simulink model "ctrl_custom"  (R2016b)
settings: Solver=ode3  StartTime=0.0  StopTime=inf  FixedStep=0.01  RelTol=1e-3  EnableMultiTasking=on
undefined symbols (not defined in the file): C, D, DiscIntNeverNeededParam, eps_c, epsilon, hd, hd2, I_s, k_cc, K_omega, K_q1f, K_q1r, K_q2f, K_q2r, K_q3f, K_q3r, K_q4f, K_q4r, K_q5f, K_q5r, K_q6f, K_q6r, K_T1f, K_T1r, K_T2f, K_T2r, K_T3f, K_T3r, K_T4f, K_T4r, K_T5f, K_T5r, K_T6f, K_T6r, Kp, Max_Acceleration, Max_rotation, Max_thrust, Min_thrust, n_c, n_max, p_cc, pwm_thr1_backward, pwm_thr1_forward, pwm_thr2_backward, pwm_thr2_forward, pwm_thr3_backward, pwm_thr3_forward, pwm_thr4_backward, pwm_thr4_forward, pwm_thr5_backward, pwm_thr5_forward, pwm_thr6_backward, pwm_thr6_forward, Q_f0, Q_max, r_cc, Rho, Thruster
libraries: dspmtrx3 x10, marine_gnc x9, simulink x7, simulink_extras x3
(part 5 of 5)

== system ctrl_custom/Thruster control /Thruster 6/Thruster control/Core controller ==
  note: Core controller: Shaft speed
  n_r : Inport
  "Tr " : Inport  Port=2
  "n " : Inport  Port=3
  Core controller: Torque,Power and Combined Torque/Power : MATLAB Function  TreatAsAtomicUnit=on
  Integrator : Integrator  ExternalReset=either  UpperSaturationLimit=Q_max  LowerSaturationLimit=-Q_max
  Ki : Gain  Gain=Kp/0.05
  Kp : Gain  Gain=Kp
  Sum : Sum  Inputs=+|-
  Sum1 : Sum  Inputs=|++
  reset : S-Function  Priority=1  FunctionName=NIVeriStandIO  Parameters=width dtype portnum stime stype btype  SFunctionDeploymentMode=off  EnableBusSupport=off  mask(NI VeriStand Inport){portnum=1, width=-1, stime=-1, dtype=auto, stype=auto, btype=1}
      mask prompts: portnum "Port number:"; width "Port dimensions (-1 for dynamically sized):"; stime "Sample time (-1 for inherited):"; dtype "Data type:"; stype "Signal type:"; btype "Block type:"
      mask help: Use this inport on any level of nested subsystems to allow NI VeriStand software to map signals to it.
      mask init:
      | NIVeriStandIO_init;
      settings: CopyFcn=NIVeriStand_MDL_functions('', 'IO_copy');  DeleteFcn=NIVeriStand_MDL_functions('', 'IO_delete');  MoveFcn=set_param(gcb, 'Mask', 'on');
      mask Callback portnum: NIVeriStand_MDL_functions('', 'IO_setportnum');
      mask TypeOptions dtype: auto | double | single | int8 | uint8 | int16 | uint16 | int32 | uint32 | boolean
      mask Callback dtype: NIVeriStand_MDL_functions('', 'IO_booleansignal');
      mask TypeOptions stype: auto | real | complex
      mask Display:
      | patch([-x x], [-y y], [.90980 .81960 .32156]);
      | plot([xrad -x x xrad], [yrad -y y yrad]);
      | fprintf('NI In%d', portnum);
  Q_cn : Outport
  Qcq : Outport  Port=2
  Qcp : Outport  Port=3
  Qcc : Outport  Port=4
  wires:
  n_r/1 -> Sum/1
  Ki/1 -> Integrator/1
  Kp/1 -> Sum1/1
  Integrator/1 -> Sum1/2
  Sum/1 -> Ki/1, Kp/1
  Sum1/1 -> Q_cn/1
  reset/1 -> Integrator/2
  [k_cc] -> Core controller: Torque,Power and Combined Torque/Power/1(k_cc)
  [p_cc] -> Core controller: Torque,Power and Combined Torque/Power/2(p_cc)
  [r_cc] -> Core controller: Torque,Power and Combined Torque/Power/3(r_cc)
  Core controller: Torque,Power and Combined Torque/Power/3(Qcc) -> Qcc/1
  [Kt6f] -> Core controller: Torque,Power and Combined Torque/Power/5(K_t0)
  [D] -> Core controller: Torque,Power and Combined Torque/Power/7(D)
  [Kq6f] -> Core controller: Torque,Power and Combined Torque/Power/6(K_q0)
  [Rho] -> Core controller: Torque,Power and Combined Torque/Power/9(rho)
  "n "/1 -> Core controller: Torque,Power and Combined Torque/Power/4(n), Sum/2
  "Tr "/1 -> Core controller: Torque,Power and Combined Torque/Power/8(Tr)
  Core controller: Torque,Power and Combined Torque/Power/2(Qcp) -> Qcp/1
  Core controller: Torque,Power and Combined Torque/Power/1(Qcq) -> Qcq/1
  [eps_c] -> Core controller: Torque,Power and Combined Torque/Power/10(eps_c)
  [Kt6r] -> Core controller: Torque,Power and Combined Torque/Power/11(K_t0r)
  [Kq6r] -> Core controller: Torque,Power and Combined Torque/Power/12(K_q0r)

== matlab function ctrl_custom/Referance/MATLAB Function ==
  data: omega input; y output; zeta input
function y = fcn(omega,zeta)

y = 2*zeta*omega;

== matlab function ctrl_custom/Referance/MATLAB Function1 ==
  data: omega input; y output; zeta input
function y = fcn(omega,zeta)

y = 2*zeta*omega;

== matlab function ctrl_custom/Referance/MATLAB Function2 ==
  data: omega input; y output
function y = fcn(omega)

y = omega*omega;

== matlab function ctrl_custom/Thrust allocation/Optimal angle path and constraints on rotation speed/Ensuring angle is [-pi pi] ==
  data: angle input; y output
function y = rad2pipi(angle)
% RAD2PIPI Converts an angle in rad to the interval (-pi pi]
%          Should be applied to all heading errors in a feedback control system
%          in order to avoid discontinuities.
%
% Author:     Roger Skjetne
% Date:       2003-09-05
% Revisions:  2004-09-02 Thor I. Fossen - replaced input argument x with angle
%             2005-01-05 Thor I. Fossen - ouput argument is set to y and not angle
%             2005-04-13 Roger Skjetne  - changed the function s in order
%                                         to account for correct mapping to
%                                         (-pi pi].
%
% ________________________________________________________________
%
% MSS GNC is a Matlab toolbox for guidance, navigation and control.
% The toolbox is part of the Marine Systems Simulator (MSS).
%
% Copyright (C) 2008 Thor I. Fossen and Tristan Perez
% 
% This program is free software: you can redistribute it and/or modify
% it under the terms of the GNU General Public License as published by
% the Free Software Foundation, either version 3 of the License, or
% (at your option) any later version.
% 
% This program is distributed in the hope that it will be useful, but
% WITHOUT ANY WARRANTY; without even the implied warranty of
% MERCHANTABILITY or FITNESS FOR A PARTICULAR PURPOSE.  See the 
% GNU General Public License for more details.
% 
% You should have received a copy of the GNU General Public License
% along with this program.  If not, see <http://www.gnu.org/licenses/>.
% 
% E-mail: contact@marinecontrol.org
% URL:    <http://www.marinecontrol.org>


% convert angle in rad to the interval <-pi pi> 
r = rem(angle+sign(angle)*pi,2*pi);
s = sign(sign(angle) + 2*(sign(abs(rem(angle+pi,2*pi)/(2*pi)))-1));
% s = sign(angle);

y = r - s*pi;

== matlab function ctrl_custom/Thruster control /Thrust and Shaft speed mapped to PWM/MATLAB Function1 ==
  data: Tc_in1 input; signal input; Tc_out output; Tc_in2 input
function Tc_out = fcn(Tc_in1,signal,Tc_in2)
%#codegen

if signal >= 0
    Tc_out = Tc_in1;
else %signal < 0
    Tc_out = Tc_in2;
end

== matlab function ctrl_custom/Thrust allocation/Optimal angle path and constraints on rotation speed/MATLAB Function1 ==
  data: desired input; psi_D output; actual input
function psi_D   = fcn(desired,actual)
%#codegen
psi_D = desired-actual;
if abs(psi_D) >= 360
    psi_D = rem(psi_D,360);
end

if abs(psi_D) >= 180
    psi_D = psi_D - sign(psi_D)*360;
end

% if desired < 0 %&& abs(desired+actual) > 180
%     y = actual+360;
% else
%     y = abs(actual);
% end

%if desired-actual > 180
%    u = desired - 360;
%elseif desired-actual <= -180
%    u=actual + 360 ;
%else
%    u=desired;        
%end

end

%rotation = change-actual;% - actual; % If positive with clock, Negative against clock
%if rotation >= 180 || rotation <= -180
% u = desired;
%else 
%     u = actual;
%end

%change = abs(actual);

% if actual-desired > 180 && desired > 0 && rotation > 0
%     u = -180;
% elseif  actual-desired > 180 && desired > 0 && rotation < 0
%     u = 180;
% else 
%     u = actual;
% end

% if change > abs(desired-actual)
%     u = -actual;
% else
%     u = actual;
% end
% if desired >= 0.98*actual || desired <= -0.98*actual 
%     u = desired;
% else 
%     u = actual; 
% end
% paths = [abs(actual-desired),abs(-1*actual-desired)];
% fastest = min(paths);
% if paths(1) > paths(2)
%     fastest = paths(2);
% elseif paths(1) < paths(2)
%     fastest = paths(1);
% end
% % if desired > 0 && actual < 0 || desired < 0 && actual < 0
% % u = fastest;
% % elseif desired > 0 && actual > 0 || desired < 0 && actual < 0
% %     u = fastest;
% if desired-actual > 180 || desired-actual < -180
%     u = -actual;
% else 
%     u = actual;
% end

== matlab function ctrl_custom/Thrust allocation/MATLAB Function ==
  data: u input; sys output; ThrusterPosX input; ThrusterPosY input; C input
function sys = fcn(u,ThrusterPosX,ThrusterPosY,C)
% Complete system goes here!
Alpha1 = zeros(1,6);    % Allocating dimensions for faster computing
% Parameters thrusters
tc =  [u(1),u(2),u(3)]'; 
alpha = [u(4),u(5),u(6),u(7),u(8),u(9)]';

% Constraints for Thruster-Thruster interaction. Can be seen in "Initfile"
% how they are found
C1 = C(1,:);
C2 = C(2,:);
C3 = C(3,:);
C4 = C(4,:);
C5 = C(5,:);
C6 = C(6,:);

K = ones(1,6);

K = ones(1,6);

if alpha(1) < C1(1)-0.1  && alpha(1) > C1(2)+0.1 || alpha(1) > C1(3)+0.1 && alpha(1) < C1(4)-0.1
    K(1) = 0;
else 
    K(1) = K(1);
end

if alpha(2) > C2(1)-0.1  && alpha(2) < C2(2)+0.1 || alpha(2) > C2(3)-0.1 && alpha(2) < C2(4)+0.1
    K(2) = 0;
else 
    K(2) = K(2);
end

if alpha(3) < C3(1)+0.1  && alpha(3) > C3(2)-0.1 || alpha(3) < C3(3)+0.1 && alpha(3) > C3(4)-0.1
    K(3) = 0;
else 
    K(3) = K(3);
end

if alpha(4) > C4(1)+0.1  && alpha(4) < C4(2)-0.1 || alpha(4) < C4(3)-0.1 && alpha(4) > C4(4)+0.1
    K(4) = 0;
else 
    K(4) = K(4);
end

if alpha(5) < C5(1)-0.1  && alpha(5) > C5(2)+0.1 || alpha(5) < C5(3)-0.1 && alpha(5) > C5(4)+0.1
    K(5) = 0;
else 
    K(5) = K(5);
end

if alpha(6) > C6(1)+0.1  && alpha(6) < C6(2)-0.1 || alpha(6) > C6(3)+0.1 && alpha(6) < C6(4)-0.1
    K(6) = 0;
else 
    K(6) = K(6);
end

epsilon = u(10);

n_t = length(ThrusterPosX); % number of thrusters
B_surge = zeros(n_t,1); % Shells for faster computing
B_sway = zeros(n_t,1);  % Shells for faster computing
B_yaw = zeros(n_t,1);   % Shells for faster computing

for i = 1:1:n_t
  B_surge(i) = cosd(alpha(i));     %Thrust in x-direction for cartesian
  B_sway(i) = sind(alpha(i));      %Thrust in y-direction for cartesian
  B_yaw(i) = (sind(alpha(i))*ThrusterPosX(i) - cosd(alpha(i))*ThrusterPosY(i));
end


B = [B_surge,B_sway,B_yaw]';
B = B*diag(K); 
[U_singular,S_singular,V_singular] = svd(B,'econ');
S_singular_cross = 1./S_singular;
S_singular_cross(~isfinite(S_singular_cross))=0;
 if (S_singular_cross(3,3)>10*S_singular_cross(2,2)) 
     S_singular_cross(3,3)=0;
 end
 
u_optimized = V_singular*S_singular_cross*U_singular';

u_d = u_optimized*tc;          % Optimized Thrust



Te = [1 0 1 0 1 0 1 0 1 0 1 0;
      0 1 0 1 0 1 0 1 0 1 0 1;
      ThrusterPosY(1) ThrusterPosX(1) ThrusterPosY(2) ThrusterPosX(2) ThrusterPosY(3) ThrusterPosX(3) ...
      ThrusterPosY(4) ThrusterPosX(4) ThrusterPosY(5) ThrusterPosX(5) ThrusterPosY(6) ThrusterPosX(6)];

[U_singular,S_singular,V_singular] = svd(Te,'econ');
S_singular_cross = 1./S_singular;
S_singular_cross(~isfinite(S_singular_cross))=0;
 if (S_singular_cross(3,3)>2*S_singular_cross(2,2)) 
     S_singular_cross(3,3)=0;
 end
T0 = V_singular*S_singular_cross*U_singular'*tc;

alpha1 = [atan2d(T0(2),T0(1)) atan2d(T0(4),T0(3)) atan2d(T0(6),T0(5)) atan2d(T0(8),T0(7)) atan2d(T0(10),T0(9)) atan2d(T0(12),T0(11))];


%% Constraints
% Thruster 1 OK
%C1 = [151 130 -151 -130 ];
if alpha1(1) < C1(1)  && alpha1(1) > C1(2) && u_d(1) > 0 || alpha1(1) < C1(1)  && alpha1(1) > C1(2) && u_d(1) < 0
    c1 = [C1(1) C1(2)];
    [C_1,alpha_new1] = min(abs(c1-alpha1(1)));
    Alpha1(1) = c1(alpha_new1);
elseif alpha1(1) > C1(3) && alpha1(1) < C1(4) && u_d(1) > 0 || alpha1(1) > C1(3) && alpha1(1) < C1(4) && u_d(1) < 0
    c1 = [C1(3) C1(4)];
    [C_1,alpha_new1] = min(abs(c1-alpha1(1)));
    Alpha1(1) = c1(alpha_new1);
else 
    Alpha1(1) = alpha1(1);
end
if alpha(1) < C1(1)-0.1  && alpha(1) > C1(2)+0.1 || alpha(1) > C1(3)+0.1 && alpha(1) < C1(4)-0.1
    u_d(1) = 0;
else 
    u_d(1) = u_d(1);
end

% Thruster 2 
%C2 = [-99.85 -80.15 -50 -29];
if alpha1(2) < C2(1)  && alpha1(2) > C2(2) && u_d(2) > 0 || alpha1(2) < C2(1)  && alpha1(2) > C2(2) && u_d(2) < 0 
    c2 = [C2(1) C2(2)];
    [C_2,alpha_new2] = min(abs(c2-alpha1(2)));
    Alpha1(2) = c2(alpha_new2);
elseif alpha1(2) < C2(3) && alpha1(2) > C2(4) && u_d(2) > 0 || alpha1(2) < C2(3) && alpha1(2) > C2(4) && u_d(2) < 0
    c2 = [C2(3) C2(4)];
    [C_2,alpha_new2] = min(abs(c2-alpha1(2)));
    Alpha1(2) = c2(alpha_new2);
else 
    Alpha1(2) = alpha1(2);
end
if alpha(2) < C2(1)-0.1  && alpha(2) > C2(2)+0.1 || alpha(2) < C2(3)-0.1 && alpha(2) > C2(4)+0.1
    u_d(2) = 0;
else 
    u_d(2) = u_d(2);
end

% Thruster 3 
% C3 = [99.85 80.15 50 29]; 

if alpha1(3) > C3(1)  && alpha1(3) < C3(2) && u_d(3) > 0 || alpha1(3) > C3(1)  && alpha1(3) < C3(2) && u_d(3) < 0
    c3 = [C3(1) C3(2)];
    [C_3,alpha_new3] = min(abs(c3-alpha1(3)));
    Alpha1(3) = c3(alpha_new3);
elseif alpha1(3) > C3(3) && alpha1(3) < C3(4) && u_d(3) > 0 || alpha1(3) > C3(3) && alpha1(3) < C3(4) && u_d(3) < 0 
    c3 = [C3(3) C3(4)];
    [C_3,alpha_new3] = min(abs(c3-alpha1(3)));
    Alpha1(3) = c3(alpha_new3);
else 
    Alpha1(3) = alpha1(3);
end
if alpha(3) > C3(1)+0.1  && alpha(3) < C3(2)-0.1 || alpha(3) > C3(3)+0.1 && alpha(3) < C3(4)-0.1
    u_d(3) = 0;
else 
    u_d(3) = u_d(3);
end

% Thruster 4 OK
%C4 = [-52.8 -34.2 52.8 34.2]; 
if alpha1(4) > C4(1)  && alpha1(4) < C4(2) && u_d(4) > 0 || alpha1(4) > C4(1)  && alpha1(4) < C4(2) && u_d(4) < 0
    c4 = [C4(1) C4(2)];
    [C_4,alpha_new4] = min(abs(c4-alpha1(4)));
    Alpha1(4) = c4(alpha_new4);
elseif alpha1(4) < C4(3) && alpha1(4) > C4(4) && u_d(4) > 0 || alpha1(4) < C4(3) && alpha1(4) > C4(4) && u_d(4) < 0 
    c4 = [C4(3) C4(4)];
    [C_4,alpha_new4] = min(abs(c4-alpha1(4)));
    Alpha1(4) = c4(alpha_new4);
else 
    Alpha1(4) = alpha1(4);
end
if alpha(4) > C4(1)+0.1  && alpha(4) < C4(2)-0.1 || alpha(4) < C4(3)-0.1 && alpha(4) > C4(4)+0.1
    u_d(4) = 0;
else 
    u_d(4) = u_d(4);
end

% Thruster 5
%C5 = [-98.25 -81.75 -145.8 -127.2];
if alpha1(5) < C5(1)  && alpha1(5) > C5(2) && u_d(5) > 0 || alpha1(5) < C5(1)  && alpha1(5) > C5(2) && u_d(5) < 0
    c5 = [C5(1) C5(2)];
    [C_5,alpha_new5] = min(abs(c5-alpha1(5)));
    Alpha1(5) = c5(alpha_new5);
elseif alpha1(5) < C5(3) && alpha1(5) > C5(4) && u_d(5) > 0  || alpha1(5) < C5(3) && alpha1(5) > C5(4) && u_d(5) < 0
    c5 = [C5(3) C5(4)];
    [C_5,alpha_new5] = min(abs(c5-alpha1(5)));
    Alpha1(5) = c5(alpha_new5);
else 
    Alpha1(5) = alpha1(5);
end
if alpha(5) < C5(1)-0.1  && alpha(5) > C5(2)+0.1 || alpha(5) < C5(3)-0.1 && alpha(5) > C5(4)+0.1
    u_d(5) = 0;
else 
    u_d(5) = u_d(5);
end

% Thruster 6
%C6 = [98.75 81.75 145.8 127.2];
if alpha1(6) > C6(1)  && alpha1(6) < C6(2) && u_d(6) > 0 || alpha1(6) > C6(1)  && alpha1(6) < C6(2) && u_d(6) < 0
    c6 = [C6(1) C6(2)];
    [C_6,alpha_new6] = min(abs(c6-alpha1(6)));
    Alpha1(6) = c6(alpha_new6);
elseif alpha1(6) > C6(3) && alpha1(6) < C6(4) && u_d(6) > 0 || alpha1(6) > C6(3) && alpha1(6) < C6(4) && u_d(6) < 0
    c6 = [C6(3) C6(4)];
    [C_6,alpha_new6] = min(abs(c6-alpha1(6)));
    Alpha1(6) = c6(alpha_new6);
else 
    Alpha1(6) = alpha1(6);
end
if alpha(6) > C6(1)+0.1  && alpha(6) < C6(2)-0.1 || alpha(6) > C6(3)+0.1 && alpha(6) < C6(4)-0.1
    u_d(6) = 0;
else 
    u_d(6) = u_d(6);
end

% Thruster 2&3 
if Alpha1(2) == C2(2)
    Alpha1(3) = alpha1(2) - (C2(2) - alpha1(2));
elseif Alpha1(2) == C2(1)
    Alpha1(3) = alpha1(2) - (C2(1) - alpha1(2));
elseif Alpha1(2) == C2(3)
    Alpha1(3) = alpha1(2) - (C2(3) - alpha1(2));
elseif Alpha1(2) == C2(4)
    Alpha1(3) = alpha1(2) - (C2(4) - alpha1(2));
    
elseif Alpha1(3) == C3(2)
    Alpha1(2) = alpha1(3) - (C3(2) - alpha1(3));
elseif Alpha1(3) == C3(1)
    Alpha1(2) = alpha1(3) - (C3(1) - alpha1(3));
elseif Alpha1(3) == C3(3)
    Alpha1(2) = alpha1(3) - (C3(3) - alpha1(3));
elseif Alpha1(3) == C3(4)
    Alpha1(2) = alpha1(3) - (C3(4) - alpha1(3));
end

% Thruster 5&6
if Alpha1(5) == C5(2)
    Alpha1(6) = alpha1(5) - (C5(2) - alpha1(5));
elseif Alpha1(5) == C5(1)
    Alpha1(6) = alpha1(5) - (C5(1) - alpha1(5));
elseif Alpha1(5) == C5(3)
    Alpha1(6) = alpha1(5) - (C5(3) - alpha1(5));
elseif Alpha1(5) == C5(4)
    Alpha1(6) = alpha1(5) - (C5(4) - alpha1(5));
    
elseif Alpha1(6) == C6(2)
    Alpha1(5) = alpha1(6) - (C6(2) - alpha1(6));
elseif Alpha1(6) == C6(1)
    Alpha1(5) = alpha1(6) - (C6(1) - alpha1(6));
elseif Alpha1(6) == C6(3)
    Alpha1(5) = alpha1(6) - (C6(3) - alpha1(6));
elseif Alpha1(6) == C6(4)
    Alpha1(5) = alpha1(6) - (C6(4) - alpha1(6));
end
% Thruster 4 & 1
if     Alpha1(4) == C4(2)
    Alpha1(1) = alpha1(4) - (C4(2) - alpha1(4));
elseif Alpha1(4) == C4(1)
    Alpha1(1) = alpha1(4) - (C4(1) - alpha1(4));
elseif Alpha1(4) == C4(3)
    Alpha1(1) = alpha1(4) - (C4(3) - alpha1(4));
elseif Alpha1(4) == C4(4)
    Alpha1(1) = alpha1(4) - (C4(4) - alpha1(4));
end

if     Alpha1(1) == C1(2)
    Alpha1(4) = alpha1(1) - (C1(2) - alpha1(1));
elseif Alpha1(1) == C1(1)
    Alpha1(4) = alpha1(1) - (C1(1) - alpha1(1));
elseif Alpha1(1) == C1(3)
    Alpha1(4) = alpha1(1) - (C1(3) - alpha1(1));
elseif Alpha1(1) == C1(4)
    Alpha1(4) = alpha1(1) - (C1(4) - alpha1(1));
end

Alpha1 = [Alpha1(1) Alpha1(2) Alpha1(3) Alpha1(4) Alpha1(5) Alpha1(6)]';    
Desired_thrust = [u_d(1) u_d(2) u_d(3) u_d(4) u_d(5) u_d(6)]';
alpha_desired = Alpha1;


% u_d = -Desired_thrust;
%% Update outputs
sys = [alpha_desired',u_d']';

== matlab function ctrl_custom/Thruster control /Thruster 1/Propeller Hydrodynamics/Actual Force and Torque ==
  data: Ta output; n input; Qa output; Kq input; Kt input; Ktr input; Kqr input; Rho input; D input; eps_c input; env input; Pa output
function [Ta,Qa,Pa]= ActualForces(n,Kq,Kt,Ktr,Kqr,Rho,D,eps_c,env)
%#codegen
lambda_c = 0.5+0.5*tanh(eps_c*n/5); % Smooth switching between positive and negative thrust. 5 makes switch happen between -5 and 5
K_TC = Kt*lambda_c+(1-lambda_c)*Ktr;
K_QC = Kq*lambda_c+(1-lambda_c)*Kqr;

Ta = sign(n)*K_TC*Rho*(D^4)*n^2-env;
Qa = sign(n)*K_QC*Rho*(D^5)*n^2-env;
Pa = 2*pi*n*Qa;

== matlab function ctrl_custom/Thruster control /Thruster 1/Thruster control/MATLAB Function ==
  data: Td input; n_d output; K_t0 input; K_t0r input; rho input; D input; eps_c input; n_c input; n_r input; T_r output
function [n_d,T_r]  = ReferenceGenerator(Td,K_t0,K_t0r,rho,D,eps_c,n_c,n_r)
%#codegen


n_d = sign(Td)*sqrt((abs(Td))/(rho*D^4*K_t0));

lambda_c = 0.5+0.5*tanh(eps_c*n_d/5); % Smooth switching between positive and negative thrust. 5 makes switch happen between -5 and 5
K_TC = K_t0*lambda_c+(1-lambda_c)*K_t0r;

T_r = sign(n_r)*K_TC*rho*D^4*n_r^2;

== matlab function ctrl_custom/Thruster control /Thruster 1/Thruster control/Supervisor ==
  data: control input; input input; n input; u output
function u = fcn(control,input,n)
u = 1;
if control == 1
if input == 1
    u = 1;
elseif input == 2
    u = 2;
elseif input == 3 && n > 0 || input == 3 && n < 0
    u = 3;
elseif input == 4 || input == 3 && n == 0
    u = 4;
else 
    u = 5;
end
end

if control == 2
if input == 1
    u = 1;
elseif input == 2
    u = 2;
elseif input == 3 && n > 0 || input == 3 && n < 0
    u = 3;
elseif input == 4 || input == 3 && n == 0
    u = 4;
else 
    u = 5;
end
end

if control == 3
if input == 1
    u = 1;
elseif input == 2
    u = 2;
elseif input == 3 && n > 0 || input == 3 && n < 0
    u = 3;
elseif input == 4 || input == 3 && n == 0
    u = 4;
else 
    u = 5;
end
end

if control == 4
if input == 1
    u = 1;
elseif input == 2
    u = 2;
elseif input == 3 && n > 0 || input == 3 && n < 0
    u = 3;
elseif input == 4 || input == 3 && n == 0
    u = 4;
else 
    u = 5;
end
end

if control == 5
if input == 1
    u = 1;
elseif input == 2
    u = 2;
elseif input == 3 && n > 0 || input == 3 && n < 0
    u = 3;
elseif input == 4 || input == 3 && n == 0
    u = 4;
else 
    u = 5;
end
end

== matlab function ctrl_custom/Thruster control /Thruster 1/Thruster control/Core controller/Core controller: Torque,Power and Combined Torque//Power ==
  data: Qcq output; Qcp output; k_cc input; p_cc input; r_cc input; n input; Qcc output; K_t0 input; K_q0 input; D input; Tr input; rho input; eps_c input; K_t0r input; K_q0r input
function [Qcq,Qcp,Qcc]= CoreControl(k_cc,p_cc,r_cc,n,K_t0,K_q0,D,Tr,rho,eps_c,K_t0r,K_q0r)
%#codegen

lambda_c = 0.5+0.5*tanh(eps_c*n/5);
K_TC = K_t0*lambda_c+(1-lambda_c)*K_t0r;
K_QC = K_q0*lambda_c+(1-lambda_c)*K_q0r;
Qcq = (K_QC/K_TC)*D*Tr;
if n == 0
    Qcp = 0;
else
Qcp = sign(Tr)*K_QC*(abs(Tr)^(3/2))/(sqrt(rho)*D*K_TC^(3/2)*abs(n));
end
alpha_c = exp(-k_cc*abs(p_cc*n)^r_cc);

Qcc = alpha_c*Qcq + (1-alpha_c)*Qcp;

== matlab function ctrl_custom/Thruster control /Thrust and Shaft speed mapped to PWM/MATLAB Function2 ==
  data: Tc_in1 input; signal input; Tc_out output; Tc_in2 input
function Tc_out = fcn(Tc_in1,signal,Tc_in2)
%#codegen

if signal >= 0
    Tc_out = Tc_in1;
else %signal < 0
    Tc_out = Tc_in2;
end

== matlab function ctrl_custom/Thruster control /Thruster 2/Propeller Hydrodynamics/Actual Force and Torque ==
  data: Ta output; n input; Qa output; Kq input; Kt input; Ktr input; Kqr input; Rho input; D input; eps_c input; env input
function [Ta,Qa]= ActualForces(n,Kq,Kt,Ktr,Kqr,Rho,D,eps_c,env)
%#codegen
lambda_c = 0.5+0.5*tanh(eps_c*n/5); % Smooth switching between positive and negative thrust. 5 makes switch happen between -5 and 5
K_TC = Kt*lambda_c+(1-lambda_c)*Ktr;
K_QC = Kq*lambda_c+(1-lambda_c)*Kqr;

Ta = sign(n)*K_TC*Rho*(D^4)*n^2-env;
Qa = sign(n)*K_QC*Rho*(D^5)*n^2-env;

== matlab function ctrl_custom/Initialization of parameters/Guidance Gains/MATLAB Function ==
  data: T_x input; y output
function y = fcn(T_x)

y = 1/T_x;

== matlab function ctrl_custom/Thrust allocation/angle between [-180 180] ==
  data: angle input; y output
function y = rad2pipi(angle)
% RAD2PIPI Converts an angle in rad to the interval (-pi pi]
%          Should be applied to all heading errors in a feedback control system
%          in order to avoid discontinuities.
%
% Author:     Roger Skjetne
% Date:       2003-09-05
% Revisions:  2004-09-02 Thor I. Fossen - replaced input argument x with angle
%             2005-01-05 Thor I. Fossen - ouput argument is set to y and not angle
%             2005-04-13 Roger Skjetne  - changed the function s in order
%                                         to account for correct mapping to
%                                         (-pi pi].
%
% ________________________________________________________________
%
% MSS GNC is a Matlab toolbox for guidance, navigation and control.
% The toolbox is part of the Marine Systems Simulator (MSS).
%
% Copyright (C) 2008 Thor I. Fossen and Tristan Perez
% 
% This program is free software: you can redistribute it and/or modify
% it under the terms of the GNU General Public License as published by
% the Free Software Foundation, either version 3 of the License, or
% (at your option) any later version.
% 
% This program is distributed in the hope that it will be useful, but
% WITHOUT ANY WARRANTY; without even the implied warranty of
% MERCHANTABILITY or FITNESS FOR A PARTICULAR PURPOSE.  See the 
% GNU General Public License for more details.
% 
% You should have received a copy of the GNU General Public License
% along with this program.  If not, see <http://www.gnu.org/licenses/>.
% 
% E-mail: contact@marinecontrol.org
% URL:    <http://www.marinecontrol.org>


% convert angle in rad to the interval <-pi pi> 
r = rem(angle+sign(angle)*pi,2*pi);
s = sign(sign(angle) + 2*(sign(abs(rem(angle+pi,2*pi)/(2*pi)))-1));
% s = sign(angle);

y = r - s*pi;

== matlab function ctrl_custom/Initialization of parameters/Guidance Gains/MATLAB Function1 ==
  data: T_y input; y output
function y = fcn(T_y)

y = 1/T_y;

== matlab function ctrl_custom/Initialization of parameters/Guidance Gains/MATLAB Function2 ==
  data: T_psi input; y output
function y = fcn(T_psi)

y = 1/T_psi;

== matlab function ctrl_custom/Thruster control /Thrust and Shaft speed mapped to PWM/MATLAB Function3 ==
  data: Tc_in1 input; signal input; Tc_out output; Tc_in2 input
function Tc_out = fcn(Tc_in1,signal,Tc_in2)
%#codegen

if signal >= 0
    Tc_out = Tc_in1;
else %signal < 0
    Tc_out = Tc_in2;
end

== matlab function ctrl_custom/Thruster control /Thruster 2/Thruster control/Core controller/Core controller: Torque,Power and Combined Torque//Power ==
  data: Qcq output; Qcp output; k_cc input; p_cc input; r_cc input; n input; Qcc output; K_t0 input; K_q0 input; D input; Tr input; rho input; eps_c input; K_t0r input; K_q0r input
function [Qcq,Qcp,Qcc]= CoreControl(k_cc,p_cc,r_cc,n,K_t0,K_q0,D,Tr,rho,eps_c,K_t0r,K_q0r)
%#codegen

lambda_c = 0.5+0.5*tanh(eps_c*n/5);
K_TC = K_t0*lambda_c+(1-lambda_c)*K_t0r;
K_QC = K_q0*lambda_c+(1-lambda_c)*K_q0r;
Qcq = (K_QC/K_TC)*D*Tr;
if n == 0
    Qcp = 0;
else
Qcp = sign(Tr)*K_QC*(abs(Tr)^(3/2))/(sqrt(rho)*D*K_TC^(3/2)*abs(n));
end
alpha_c = exp(-k_cc*abs(p_cc*n)^r_cc);

Qcc = alpha_c*Qcq + (1-alpha_c)*Qcp;

== matlab function ctrl_custom/Thruster control /Thruster 2/Thruster control/MATLAB Function ==
  data: Td input; n_d output; K_t0 input; K_t0r input; rho input; D input; eps_c input; n_c input; n_r input; T_r output
function [n_d,T_r]  = ReferenceGenerator(Td,K_t0,K_t0r,rho,D,eps_c,n_c,n_r)
%#codegen


n_d = sign(Td)*sqrt((abs(Td))/(rho*D^4*K_t0));

lambda_c = 0.5+0.5*tanh(eps_c*n_d/5); % Smooth switching between positive and negative thrust
K_TC = K_t0*lambda_c+(1-lambda_c)*K_t0r;

T_r = sign(n_r)*K_TC*rho*D^4*n_r^2;

== matlab function ctrl_custom/Thruster control /Thruster 2/Thruster control/Supervisor ==
  data: control input; input input; n input; u output
function u = fcn(control,input,n)
u = 1;
if control == 1
if input == 1
    u = 1;
elseif input == 2
    u = 2;
elseif input == 3 && n > 0 || input == 3 && n < 0
    u = 3;
elseif input == 4 || input == 3 && n == 0
    u = 4;
else 
    u = 5;
end
end

if control == 2
if input == 1
    u = 1;
elseif input == 2
    u = 2;
elseif input == 3 && n > 0 || input == 3 && n < 0
    u = 3;
elseif input == 4 || input == 3 && n == 0
    u = 4;
else 
    u = 5;
end
end

if control == 3
if input == 1
    u = 1;
elseif input == 2
    u = 2;
elseif input == 3 && n > 0 || input == 3 && n < 0
    u = 3;
elseif input == 4 || input == 3 && n == 0
    u = 4;
else 
    u = 5;
end
end

if control == 4
if input == 1
    u = 1;
elseif input == 2
    u = 2;
elseif input == 3 && n > 0 || input == 3 && n < 0
    u = 3;
elseif input == 4 || input == 3 && n == 0
    u = 4;
else 
    u = 5;
end
end

if control == 5
if input == 1
    u = 1;
elseif input == 2
    u = 2;
elseif input == 3 && n > 0 || input == 3 && n < 0
    u = 3;
elseif input == 4 || input == 3 && n == 0
    u = 4;
else 
    u = 5;
end
end

== matlab function ctrl_custom/Thruster control /Thrust and Shaft speed mapped to PWM/MATLAB Function4 ==
  data: Tc_in1 input; signal input; Tc_out output; Tc_in2 input
function Tc_out = fcn(Tc_in1,signal,Tc_in2)
%#codegen

if signal >= 0
    Tc_out = Tc_in1;
else %signal < 0
    Tc_out = Tc_in2;
end

== matlab function ctrl_custom/Thruster control /Thruster 3/Propeller Hydrodynamics/Actual Force and Torque ==
  data: Ta output; n input; Qa output; Kq input; Kt input; Ktr input; Kqr input; Rho input; D input; eps_c input; env input
function [Ta,Qa]= ActualForces(n,Kq,Kt,Ktr,Kqr,Rho,D,eps_c,env)
%#codegen
lambda_c = 0.5+0.5*tanh(eps_c*n/5); % Smooth switching between positive and negative thrust. 5 makes switch happen between -5 and 5
K_TC = Kt*lambda_c+(1-lambda_c)*Ktr;
K_QC = Kq*lambda_c+(1-lambda_c)*Kqr;

Ta = sign(n)*K_TC*Rho*(D^4)*n^2-env;
Qa = sign(n)*K_QC*Rho*(D^5)*n^2-env;

== matlab function ctrl_custom/MATLAB Function ==
  data: thrust_actual input; commanded_tau output; alpha_actual input; PosX input; PosY input
function commanded_tau   = fcn(thrust_actual,alpha_actual,PosX,PosY)
%#codegen

Alpha_surge =[cosd(alpha_actual(1)) cosd(alpha_actual(2)) cosd(alpha_actual(3)) cosd(alpha_actual(4)) cosd(alpha_actual(5)) cosd(alpha_actual(6))];  
Alpha_sway = [sind(alpha_actual(1)) sind(alpha_actual(2)) sind(alpha_actual(3)) sind(alpha_actual(4)) sind(alpha_actual(5)) sind(alpha_actual(6))];
Alpha_yaw = [sind(alpha_actual(1))*PosX(1)-cosd(alpha_actual(1))*PosY(1) sind(alpha_actual(2))*PosX(2)-cosd(alpha_actual(2))*PosY(2) ...
             sind(alpha_actual(3))*PosX(3)-cosd(alpha_actual(3))*PosY(3) sind(alpha_actual(4))*PosX(4)-cosd(alpha_actual(4))*PosY(4) ...
             sind(alpha_actual(5))*PosX(5)-cosd(alpha_actual(5))*PosY(5) sind(alpha_actual(6))*PosX(6)-cosd(alpha_actual(6))*PosY(6)];

commanded_tau = [Alpha_surge;Alpha_sway;Alpha_yaw]*thrust_actual;

== matlab function ctrl_custom/Thruster control /Thrust and Shaft speed mapped to PWM/MATLAB Function5 ==
  data: Tc_in1 input; signal input; Tc_out output; Tc_in2 input
function Tc_out = fcn(Tc_in1,signal,Tc_in2)
%#codegen

if signal >= 0
    Tc_out = Tc_in1;
else %signal < 0
    Tc_out = Tc_in2;
end

== matlab function ctrl_custom/Thruster control /Thruster 3/Thruster control/Core controller/Core controller: Torque,Power and Combined Torque//Power ==
  data: Qcq output; Qcp output; k_cc input; p_cc input; r_cc input; n input; Qcc output; K_t0 input; K_q0 input; D input; Tr input; rho input; eps_c input; K_t0r input; K_q0r input
function [Qcq,Qcp,Qcc]= CoreControl(k_cc,p_cc,r_cc,n,K_t0,K_q0,D,Tr,rho,eps_c,K_t0r,K_q0r)
%#codegen

lambda_c = 0.5+0.5*tanh(eps_c*n/5);
K_TC = K_t0*lambda_c+(1-lambda_c)*K_t0r;
K_QC = K_q0*lambda_c+(1-lambda_c)*K_q0r;
Qcq = (K_QC/K_TC)*D*Tr;
if n == 0
    Qcp = 0;
else
Qcp = sign(Tr)*K_QC*(abs(Tr)^(3/2))/(sqrt(rho)*D*K_TC^(3/2)*abs(n));
end
alpha_c = exp(-k_cc*abs(p_cc*n)^r_cc);

Qcc = alpha_c*Qcq + (1-alpha_c)*Qcp;

== matlab function ctrl_custom/Thruster control /Thruster 3/Thruster control/MATLAB Function ==
  data: Td input; n_d output; K_t0 input; K_t0r input; rho input; D input; eps_c input; n_c input; n_r input; T_r output
function [n_d,T_r]  = ReferenceGenerator(Td,K_t0,K_t0r,rho,D,eps_c,n_c,n_r)
%#codegen


n_d = sign(Td)*sqrt((abs(Td))/(rho*D^4*K_t0));

lambda_c = 0.5+0.5*tanh(eps_c*n_d/5); % Smooth switching between positive and negative thrust
K_TC = K_t0*lambda_c+(1-lambda_c)*K_t0r;

T_r = sign(n_r)*K_TC*rho*D^4*n_r^2;

== matlab function ctrl_custom/Thruster control /Thrust and Shaft speed mapped to PWM/MATLAB Function ==
  data: input input; output output; control input; speedcontrol input
function output = fcn(input,control,speedcontrol)
%#codegen
if control == 1
output = [input(1) speedcontrol(1) input(3) speedcontrol(2) input(5) speedcontrol(3) input(7) speedcontrol(4) input(9) speedcontrol(5) input(11) speedcontrol(6)]';
%     output = [input(1) input(2) input(3) input(4) input(5) input(6) input(7) input(8) input(9) input(10) input(11) input(12)]';

else
    output = [input(1) input(2) input(3) input(4) input(5) input(6) input(7) input(8) input(9) input(10) input(11) input(12)]';

end

== matlab function ctrl_custom/Thruster control /Thrust and Shaft speed mapped to PWM/MATLAB Function6 ==
  data: Tc_in1 input; signal input; Tc_out output; Tc_in2 input
function Tc_out = fcn(Tc_in1,signal,Tc_in2)
%#codegen

if signal >= 0
    Tc_out = Tc_in1;
else %signal < 0
    Tc_out = Tc_in2;
end

== matlab function ctrl_custom/Initialization of parameters/Setpoint Chasing/MATLAB Function ==
  data: Ts_x input; y output
function y = fcn(Ts_x)

Ts_x_model = Ts_x/sqrt(90);

y = 1/Ts_x_model;

== matlab function ctrl_custom/Initialization of parameters/Setpoint Chasing/MATLAB Function1 ==
  data: Ts_y input; y output
function y = fcn(Ts_y)

Ts_y_model = Ts_y/sqrt(90);

y = 1/Ts_y_model;

== matlab function ctrl_custom/Thruster control /Thruster 3/Thruster control/Supervisor ==
  data: control input; input input; n input; u output
function u = fcn(control,input,n)
u = 1;
if control == 1
if input == 1
    u = 1;
elseif input == 2
    u = 2;
elseif input == 3 && n > 0 || input == 3 && n < 0
    u = 3;
elseif input == 4 || input == 3 && n == 0
    u = 4;
else 
    u = 5;
end
end

if control == 2
if input == 1
    u = 1;
elseif input == 2
    u = 2;
elseif input == 3 && n > 0 || input == 3 && n < 0
    u = 3;
elseif input == 4 || input == 3 && n == 0
    u = 4;
else 
    u = 5;
end
end

if control == 3
if input == 1
    u = 1;
elseif input == 2
    u = 2;
elseif input == 3 && n > 0 || input == 3 && n < 0
    u = 3;
elseif input == 4 || input == 3 && n == 0
    u = 4;
else 
    u = 5;
end
end

if control == 4
if input == 1
    u = 1;
elseif input == 2
    u = 2;
elseif input == 3 && n > 0 || input == 3 && n < 0
    u = 3;
elseif input == 4 || input == 3 && n == 0
    u = 4;
else 
    u = 5;
end
end

if control == 5
if input == 1
    u = 1;
elseif input == 2
    u = 2;
elseif input == 3 && n > 0 || input == 3 && n < 0
    u = 3;
elseif input == 4 || input == 3 && n == 0
    u = 4;
else 
    u = 5;
end
end

== matlab function ctrl_custom/Thruster control /Thruster 4/Propeller Hydrodynamics/Actual Force and Torque ==
  data: Ta output; n input; Qa output; Kq input; Kt input; Ktr input; Kqr input; Rho input; D input; eps_c input; env input
function [Ta,Qa]= ActualForces(n,Kq,Kt,Ktr,Kqr,Rho,D,eps_c,env)
%#codegen
lambda_c = 0.5+0.5*tanh(eps_c*n/5); % Smooth switching between positive and negative thrust. 5 makes switch happen between -5 and 5
K_TC = Kt*lambda_c+(1-lambda_c)*Ktr;
K_QC = Kq*lambda_c+(1-lambda_c)*Kqr;

Ta = sign(n)*K_TC*Rho*(D^4)*n^2-env;
Qa = sign(n)*K_QC*Rho*(D^5)*n^2-env;

== matlab function ctrl_custom/Thruster control /Thruster 4/Thruster control/Core controller/Core controller: Torque,Power and Combined Torque//Power ==
  data: Qcq output; Qcp output; k_cc input; p_cc input; r_cc input; n input; Qcc output; K_t0 input; K_q0 input; D input; Tr input; rho input; eps_c input; K_t0r input; K_q0r input
function [Qcq,Qcp,Qcc]= CoreControl(k_cc,p_cc,r_cc,n,K_t0,K_q0,D,Tr,rho,eps_c,K_t0r,K_q0r)
%#codegen

lambda_c = 0.5+0.5*tanh(eps_c*n/5);
K_TC = K_t0*lambda_c+(1-lambda_c)*K_t0r;
K_QC = K_q0*lambda_c+(1-lambda_c)*K_q0r;
Qcq = (K_QC/K_TC)*D*Tr;
if n == 0
    Qcp = 0;
else
Qcp = sign(Tr)*K_QC*(abs(Tr)^(3/2))/(sqrt(rho)*D*K_TC^(3/2)*abs(n));
end
alpha_c = exp(-k_cc*abs(p_cc*n)^r_cc);

Qcc = alpha_c*Qcq + (1-alpha_c)*Qcp;

== matlab function ctrl_custom/Thruster control /Thruster 4/Thruster control/MATLAB Function ==
  data: Td input; n_d output; K_t0 input; K_t0r input; rho input; D input; eps_c input; n_c input; n_r input; T_r output
function [n_d,T_r]  = ReferenceGenerator(Td,K_t0,K_t0r,rho,D,eps_c,n_c,n_r)
%#codegen


n_d = sign(Td)*sqrt((abs(Td))/(rho*D^4*K_t0));

lambda_c = 0.5+0.5*tanh(eps_c*n_d/5); % Smooth switching between positive and negative thrust
K_TC = K_t0*lambda_c+(1-lambda_c)*K_t0r;

T_r = sign(n_r)*K_TC*rho*D^4*n_r^2;

== matlab function ctrl_custom/Thruster control /Thruster 4/Thruster control/Supervisor ==
  data: control input; input input; n input; u output
function u = fcn(control,input,n)
u = 1;
if control == 1
if input == 1
    u = 1;
elseif input == 2
    u = 2;
elseif input == 3 && n > 0 || input == 3 && n < 0
    u = 3;
elseif input == 4 || input == 3 && n == 0
    u = 4;
else 
    u = 5;
end
end

if control == 2
if input == 1
    u = 1;
elseif input == 2
    u = 2;
elseif input == 3 && n > 0 || input == 3 && n < 0
    u = 3;
elseif input == 4 || input == 3 && n == 0
    u = 4;
else 
    u = 5;
end
end

if control == 3
if input == 1
    u = 1;
elseif input == 2
    u = 2;
elseif input == 3 && n > 0 || input == 3 && n < 0
    u = 3;
elseif input == 4 || input == 3 && n == 0
    u = 4;
else 
    u = 5;
end
end

if control == 4
if input == 1
    u = 1;
elseif input == 2
    u = 2;
elseif input == 3 && n > 0 || input == 3 && n < 0
    u = 3;
elseif input == 4 || input == 3 && n == 0
    u = 4;
else 
    u = 5;
end
end

if control == 5
if input == 1
    u = 1;
elseif input == 2
    u = 2;
elseif input == 3 && n > 0 || input == 3 && n < 0
    u = 3;
elseif input == 4 || input == 3 && n == 0
    u = 4;
else 
    u = 5;
end
end

== matlab function ctrl_custom/Thruster control /Thruster 5/Propeller Hydrodynamics/Actual Force and Torque ==
  data: Ta output; n input; Qa output; Kq input; Kt input; Ktr input; Kqr input; Rho input; D input; eps_c input; env input
function [Ta,Qa]= ActualForces(n,Kq,Kt,Ktr,Kqr,Rho,D,eps_c,env)
%#codegen
lambda_c = 0.5+0.5*tanh(eps_c*n/5); % Smooth switching between positive and negative thrust. 5 makes switch happen between -5 and 5
K_TC = Kt*lambda_c+(1-lambda_c)*Ktr;
K_QC = Kq*lambda_c+(1-lambda_c)*Kqr;

Ta = sign(n)*K_TC*Rho*(D^4)*n^2-env;
Qa = sign(n)*K_QC*Rho*(D^5)*n^2-env;

== matlab function ctrl_custom/Thruster control /Thruster 5/Thruster control/Core controller/Core controller: Torque,Power and Combined Torque//Power ==
  data: Qcq output; Qcp output; k_cc input; p_cc input; r_cc input; n input; Qcc output; K_t0 input; K_q0 input; D input; Tr input; rho input; eps_c input; K_t0r input; K_q0r input
function [Qcq,Qcp,Qcc]= CoreControl(k_cc,p_cc,r_cc,n,K_t0,K_q0,D,Tr,rho,eps_c,K_t0r,K_q0r)
%#codegen

lambda_c = 0.5+0.5*tanh(eps_c*n/5);
K_TC = K_t0*lambda_c+(1-lambda_c)*K_t0r;
K_QC = K_q0*lambda_c+(1-lambda_c)*K_q0r;
Qcq = (K_QC/K_TC)*D*Tr;
if n == 0
    Qcp = 0;
else
Qcp = sign(Tr)*K_QC*(abs(Tr)^(3/2))/(sqrt(rho)*D*K_TC^(3/2)*abs(n));
end
alpha_c = exp(-k_cc*abs(p_cc*n)^r_cc);

Qcc = alpha_c*Qcq + (1-alpha_c)*Qcp;

== matlab function ctrl_custom/Thruster control /Thruster 5/Thruster control/MATLAB Function ==
  data: Td input; n_d output; K_t0 input; K_t0r input; rho input; D input; eps_c input; n_c input; n_r input; T_r output
function [n_d,T_r]  = ReferenceGenerator(Td,K_t0,K_t0r,rho,D,eps_c,n_c,n_r)
%#codegen


n_d = sign(Td)*sqrt((abs(Td))/(rho*D^4*K_t0));

lambda_c = 0.5+0.5*tanh(eps_c*n_d/5); % Smooth switching between positive and negative thrust
K_TC = K_t0*lambda_c+(1-lambda_c)*K_t0r;

T_r = sign(n_r)*K_TC*rho*D^4*n_r^2;

== matlab function ctrl_custom/Thruster control /Thruster 5/Thruster control/Supervisor ==
  data: control input; input input; n input; u output
function u = fcn(control,input,n)
u = 1;
if control == 1
if input == 1
    u = 1;
elseif input == 2
    u = 2;
elseif input == 3 && n > 0 || input == 3 && n < 0
    u = 3;
elseif input == 4 || input == 3 && n == 0
    u = 4;
else 
    u = 5;
end
end

if control == 2
if input == 1
    u = 1;
elseif input == 2
    u = 2;
elseif input == 3 && n > 0 || input == 3 && n < 0
    u = 3;
elseif input == 4 || input == 3 && n == 0
    u = 4;
else 
    u = 5;
end
end

if control == 3
if input == 1
    u = 1;
elseif input == 2
    u = 2;
elseif input == 3 && n > 0 || input == 3 && n < 0
    u = 3;
elseif input == 4 || input == 3 && n == 0
    u = 4;
else 
    u = 5;
end
end

if control == 4
if input == 1
    u = 1;
elseif input == 2
    u = 2;
elseif input == 3 && n > 0 || input == 3 && n < 0
    u = 3;
elseif input == 4 || input == 3 && n == 0
    u = 4;
else 
    u = 5;
end
end

if control == 5
if input == 1
    u = 1;
elseif input == 2
    u = 2;
elseif input == 3 && n > 0 || input == 3 && n < 0
    u = 3;
elseif input == 4 || input == 3 && n == 0
    u = 4;
else 
    u = 5;
end
end

== matlab function ctrl_custom/Thruster control /Thruster 6/Propeller Hydrodynamics/Actual Force and Torque ==
  data: Ta output; n input; Qa output; Kq input; Kt input; Ktr input; Kqr input; Rho input; D input; eps_c input; env input
function [Ta,Qa]= ActualForces(n,Kq,Kt,Ktr,Kqr,Rho,D,eps_c,env)
%#codegen
lambda_c = 0.5+0.5*tanh(eps_c*n/5); % Smooth switching between positive and negative thrust. 5 makes switch happen between -5 and 5
K_TC = Kt*lambda_c+(1-lambda_c)*Ktr;
K_QC = Kq*lambda_c+(1-lambda_c)*Kqr;

Ta = sign(n)*K_TC*Rho*(D^4)*n^2-env;
Qa = sign(n)*K_QC*Rho*(D^5)*n^2-env;

== matlab function ctrl_custom/Thruster control /Thruster 6/Thruster control/Core controller/Core controller: Torque,Power and Combined Torque//Power ==
  data: Qcq output; Qcp output; k_cc input; p_cc input; r_cc input; n input; Qcc output; K_t0 input; K_q0 input; D input; Tr input; rho input; eps_c input; K_t0r input; K_q0r input
function [Qcq,Qcp,Qcc]= CoreControl(k_cc,p_cc,r_cc,n,K_t0,K_q0,D,Tr,rho,eps_c,K_t0r,K_q0r)
%#codegen

lambda_c = 0.5+0.5*tanh(eps_c*n/5);
K_TC = K_t0*lambda_c+(1-lambda_c)*K_t0r;
K_QC = K_q0*lambda_c+(1-lambda_c)*K_q0r;
Qcq = (K_QC/K_TC)*D*Tr;
if n == 0
    Qcp = 0;
else
Qcp = sign(Tr)*K_QC*(abs(Tr)^(3/2))/(sqrt(rho)*D*K_TC^(3/2)*abs(n));
end
alpha_c = exp(-k_cc*abs(p_cc*n)^r_cc);

Qcc = alpha_c*Qcq + (1-alpha_c)*Qcp;

== matlab function ctrl_custom/Thruster control /Thruster 6/Thruster control/MATLAB Function ==
  data: Td input; n_d output; K_t0 input; K_t0r input; rho input; D input; eps_c input; n_c input; n_r input; T_r output
function [n_d,T_r]  = ReferenceGenerator(Td,K_t0,K_t0r,rho,D,eps_c,n_c,n_r)
%#codegen


n_d = sign(Td)*sqrt((abs(Td))/(rho*D^4*K_t0));

lambda_c = 0.5+0.5*tanh(eps_c*n_d/27); % Smooth switching between positive and negative thrust
K_TC = K_t0*lambda_c+(1-lambda_c)*K_t0r;

T_r = sign(n_r)*K_TC*rho*D^4*n_r^2;

== matlab function ctrl_custom/Thruster control /Thruster 6/Thruster control/Supervisor ==
  data: control input; input input; n input; u output
function u = fcn(control,input,n)
u = 1;
if control == 1
if input == 1
    u = 1;
elseif input == 2
    u = 2;
elseif input == 3 && n > 0 || input == 3 && n < 0
    u = 3;
elseif input == 4 || input == 3 && n == 0
    u = 4;
else 
    u = 5;
end
end

if control == 2
if input == 1
    u = 1;
elseif input == 2
    u = 2;
elseif input == 3 && n > 0 || input == 3 && n < 0
    u = 3;
elseif input == 4 || input == 3 && n == 0
    u = 4;
else 
    u = 5;
end
end

if control == 3
if input == 1
    u = 1;
elseif input == 2
    u = 2;
elseif input == 3 && n > 0 || input == 3 && n < 0
    u = 3;
elseif input == 4 || input == 3 && n == 0
    u = 4;
else 
    u = 5;
end
end

if control == 4
if input == 1
    u = 1;
elseif input == 2
    u = 2;
elseif input == 3 && n > 0 || input == 3 && n < 0
    u = 3;
elseif input == 4 || input == 3 && n == 0
    u = 4;
else 
    u = 5;
end
end

if control == 5
if input == 1
    u = 1;
elseif input == 2
    u = 2;
elseif input == 3 && n > 0 || input == 3 && n < 0
    u = 3;
elseif input == 4 || input == 3 && n == 0
    u = 4;
else 
    u = 5;
end
end

== matlab function ctrl_custom/Nonlinear Passisve Observer/C(nu)*nu ==
  data: nu_hat input; C_nl output
function C_nl = fcn(nu_hat)
%#codegen
u = nu_hat(1);
v = nu_hat(2);
r = nu_hat(3);

%% MATRICES
m    = 127.92;   x_g = 0; %0.0432;

%% Added mass
X_ud  =   3.262;	Y_vd =      28.89;		Y_rd =      0.525;

%% Correolis matrix
c_13 = -(m-Y_vd)*v-(m*x_g-Y_rd)*r;
c_23 = (m-X_ud)*u;

C    = [0     0     c_13
        0     0     c_23
        -c_13 -c_23 0   ];

    
C_NL = C;

C_nl =C_NL*nu_hat;

== matlab function ctrl_custom/Nonlinear Passisve Observer/D(nu)*nu ==
  data: nu_hat input; D_nl output
function D_nl = fcn(nu_hat)
%#codegen
u = nu_hat(1);
v = nu_hat(2);
r = nu_hat(3);

%% DAMPING 

% Surge:
% Based on fitting of towing data from -0.8 < u < 0.8 m/s
X_u     = -2.332;
X_uu	=  0;
X_uuu	= -8.557;

% Sway:
% Based on fitting of towing data from -0.45 < u < 0.45 m/s
Y_v 	= -4.673;
Y_vv	=  0.3976;
Y_vvv	= -313.3;

% Yaw:
% Based on fitting of towing data from -8 < u < 8 deg/s
% The fitting range is limited. Towing should be performed for higher
% velocities.
N_r		= -0.01675;
N_rr	= -0.01148;
N_rrr	= -0.0003578;

% Y_vvv og N_rrr er fra curvefitting uten minus, men ser ut til å fungere
% med minus. 
                           N_v		= 0;                Y_r	    =  -7.250; 
                           N_vv	    = -0.2088;          Y_rr	=  -3.450;
                           N_vvv	= 0;                Y_rrr	=  0;
						
						   Y_rv	    = -0.805;			Y_vr	=  -0.845; 

						   N_rv	    = 0.08;             N_vr	= 0.08;
                           
%% Assembly of the damping matrix
d_11 = X_u + X_uu*abs(u) + X_uuu*u^2;
d_22 = Y_v + Y_vv*abs(v) + Y_vvv*v^2;
d_33 = N_r + N_rr*abs(r) + N_rrr*r^2;

d_23 = 0; % Y_r + Y_rr*abs(r) + Y_rrr*r^2 + Y_vr*abs(v); Not verified, temporarily disabled
d_32 = 0; % N_v + N_vv*abs(v) + N_vvv*v^2 + N_rv*abs(r); Not verified, temporarily disabled

D    = - [d_11 0    0
          0    d_22 d_23
          0    d_32 d_33];


D_NL = D;

D_nl =D_NL*nu_hat;
